simulink model "mbk"  (R2018a)
settings: Solver=ode4  StartTime=0.0  StopTime=50  FixedStep=0.01  RelTol=1e-3
values from neighbouring files (symbols this model uses):
  b = 2    [Kalman.m]    (also in fcn.m = 5; untitled2.m = 5)
  k = 2    [Kalman.m]    (also in fcn.m = 5; temtProp.m = 100; untitled2.m = 5)
  m = 10    [Kalman.m]    (also in fcn.m; temtProp.m; untitled2.m)
settings Model: Creator=Ali  LastModifiedBy=Ali

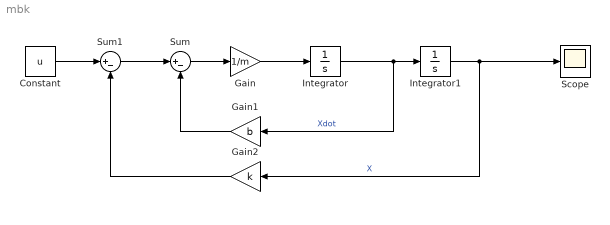
== system mbk ==
  Constant : Constant  Value=u
  Gain : Gain  Gain=1/m
  Gain1 : Gain  Gain=b
  Gain2 : Gain  Gain=k
  Integrator : Integrator
  Integrator1 : Integrator  InitialCondition=10
  Scope : Scope
  Sum : Sum  Inputs=|+-
  Sum1 : Sum  Inputs=|+-
  wires:
  Integrator/1 -> Gain1/1, Integrator1/1  "Xdot"
  Integrator1/1 -> Gain2/1, Scope/1  "X"
  Gain/1 -> Integrator/1
  Sum/1 -> Gain/1
  Gain1/1 -> Sum/2
  Sum1/1 -> Sum/1
  Gain2/1 -> Sum1/2
  Constant/1 -> Sum1/1
